simulink model "Demo_M1V4_9250"  (R2015a)
settings: Solver=FixedStepDiscrete  SolverMode=SingleTasking  StartTime=0.0  StopTime=inf  FixedStep=.03  RelTol=1e-3
libraries: RASPlib x7, MinSegLibrary_M1V4 x4, arduinolib x3
settings Model: SimulationMode=external  ExtModeTrigDuration=2  Creator=Alec  LastModifiedBy=hurstj
settings OptimizationCC: ExpressionDepthLimit=2147483647  OptimizeModelRefInitCode=on  LifeSpan=1
settings DebuggingCC: UnderspecifiedInitializationDetection=Classic  MergeDetectMultiDrivingBlocksExec=none  StateNameClashWarn=warning
settings HardwareCC: ProdBitPerInt=16  ProdBitPerPointer=8  ProdIntDivRoundTo=Zero  ProdEndianess=LittleEndian  ProdWordSize=8  ProdHWDeviceType=Atmel->AVR
settings RTWCC: SystemTargetFile=realtime.tlc  GenerateMakefile=off  TemplateMakefile=realtime.tmf  Description=Real-Time Toolbox  RTWVerbose=off
settings CodeAppCC: CustomSymbolStrType=$N$R$M  InternalIdentifier=Classic
settings ERTTargetCC: CombineOutputUpdateFcns=off  ExtMode=on  ExtModeTransport=3  ExtModeMexArgs=0 4 115200 30  ERTSrcFileBannerTemplate=realtime_code_template.cgt  ERTHdrFileBannerTemplate=realtime_code_template.cgt  ERTDataSrcFileTemplate=realtime_code_template.cgt  ERTDataHdrFileTemplate=realtime_code_template.cgt  ERTCustomFileTemplate=realtime_file_process.tlc

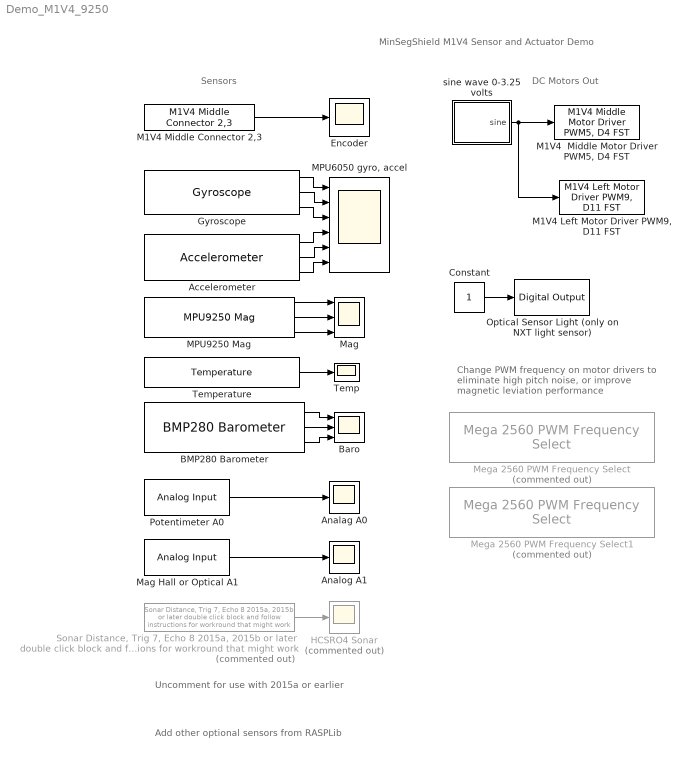
== system Demo_M1V4_9250 ==
  note: Add other optional sensors from RASPLib
  note: Uncomment for use with 2015a or earlier
  note: DC Motors Out
  note: Sensors
  note: MinSegShield M1V4 Sensor and Actuator Demo
  note: Change PWM frequency on motor drivers
      | to eliminate high pitch noise, or improve
      | magnetic leviation performance
  Accelerometer : RASPlib/Accelerometer  SimulateUsing=Code generation
  Analag A0 : Scope
      settings: TimeRange=30  YMin=200  YMax=1100  SaveName=ScopeData6
  Analog A1 : Scope
      settings: TimeRange=30  YMin=200  YMax=1100  SaveName=ScopeData3
  BMP280 Barometer : RASPlib/BMP280 Barometer  SimulateUsing=Code generation
  Baro : Scope  NumInputPorts=3
      settings: TimeRange=10  YMin=-1~44330~27.7  YMax=1~44330~28.2  SaveName=ScopeData4
  Constant : Constant
  Encoder : Scope
      settings: TimeRange=10  YMin=-50  YMax=750
  Gyroscope : RASPlib/Gyroscope  DLPFmode=0
  HCSRO4 Sonar : Scope  Commented=on
      settings: TimeRange=30  YMin=0  YMax=150  SaveName=ScopeData2
  "M1V4  Middle Motor Driver PWM5, D4 FST" : MinSegLibrary_M1V4/M1V4  Middle Motor Driver PWM5, D4 FST  Vsupply=3.25
  "M1V4 Left Motor Driver PWM9, D11 FST" : MinSegLibrary_M1V4/M1V4 Left Motor Driver PWM9, D11 FST  Vsupply=3.25
  M1V4 Middle Connector 2,3 : MinSegLibrary_M1V4/M1V4 Middle Connector 2,3  Encoder=0  PinA=3  PinB=2
  "MPU6050 gyro, accel" : Scope  NumInputPorts=6
      settings: TimeRange=10  YMin=-40000~-40000~-40000~-25000~-10000~-15000  YMax=40000~40000~40000~20000~12500~35000
  MPU9250 Mag : RASPlib/MPU9250 Mag  SimulateUsing=Code generation
  Mag : Scope  NumInputPorts=3
      settings: TimeRange=10  YMin=-200~-200~-200  YMax=200~200~200  SaveName=ScopeData7
  Mag Hall or Optical A1 : arduinolib/Analog Input  pinNumber=1  sampleTime=-1  blockPlatform=arduino
  Mega 2560 PWM Frequency Select : RASPlib/Mega 2560 PWM Frequency Select  Commented=on  Frequency=32KHz  Timer=2 - pins 9, 10
  Mega 2560 PWM Frequency Select1 : RASPlib/Mega 2560 PWM Frequency Select  Commented=on  Frequency=32KHz  Timer=3 - pins 2, 3, 5
  Optical Sensor Light (only on NXT light sensor) : arduinolib/Digital Output  pinNumber=12  blockPlatform=arduino
  Potentimeter A0 : arduinolib/Analog Input  pinNumber=0  sampleTime=-1  blockPlatform=arduino
  "Sonar Distance, Trig 7, Echo 8 2015a, 2015b or later double click block and follow instructions for workround that might work" : MinSegLibrary_M1V4/Sonar Distance, Trig 7, Echo 8 2015a, 2015b or later double click block and follow instructions for workround that might work  Commented=on  Sonar=1  TrigPin=7  EchoPin=8
  Temp : Scope
      settings: TimeRange=30  YMin=1500  YMax=1650  SaveName=ScopeData9
  Temperature : RASPlib/Temperature  SimulateUsing=Code generation
  sine wave 0-3.25 volts : Subsystem
  wires:
  sine wave 0-3.25 volts/1(sine) -> "M1V4 Left Motor Driver PWM9, D11 FST"/1, "M1V4  Middle Motor Driver PWM5, D4 FST"/1
  Potentimeter A0/1 -> Analag A0/1
  Mag Hall or Optical A1/1 -> Analog A1/1
  Constant/1 -> Optical Sensor Light (only on NXT light sensor)/1
  M1V4 Middle Connector 2,3/1 -> Encoder/1
  "Sonar Distance, Trig 7, Echo 8 2015a, 2015b or later double click block and follow instructions for workround that might work"/1 -> HCSRO4 Sonar/1
  Gyroscope/2 -> "MPU6050 gyro, accel"/2
  Gyroscope/3 -> "MPU6050 gyro, accel"/3
  Accelerometer/1 -> "MPU6050 gyro, accel"/4
  Accelerometer/2 -> "MPU6050 gyro, accel"/5
  Accelerometer/3 -> "MPU6050 gyro, accel"/6
  MPU9250 Mag/1 -> Mag/1
  MPU9250 Mag/2 -> Mag/2
  MPU9250 Mag/3 -> Mag/3
  Temperature/1 -> Temp/1
  Gyroscope/1 -> "MPU6050 gyro, accel"/1
  BMP280 Barometer/1 -> Baro/1
  BMP280 Barometer/2 -> Baro/2
  BMP280 Barometer/3 -> Baro/3

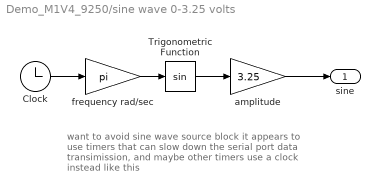
== system Demo_M1V4_9250/sine wave 0-3.25 volts ==
  note: want to avoid sine wave source block
      | it appears to use timers that can slow down the
      | serial port data transimission, and maybe
      | other timers
      |
      | use a clock instead like this
  Clock : Clock
  Trigonometric Function : Trigonometry
  amplitude : Gain  Gain=3.25
  frequency rad/sec : Gain  Gain=pi
  sine : Outport
  wires:
  Clock/1 -> frequency rad/sec/1
  Trigonometric Function/1 -> amplitude/1
  frequency rad/sec/1 -> Trigonometric Function/1
  amplitude/1 -> sine/1
